simulink model "acf_detector_sl"  (R2018b)
settings: Solver=FixedStepDiscrete  StartTime=0.0  StopTime=inf  FixedStep=0.5  RelTol=1e-3
model workspace (MAT data in the model file):
  SL_ROS_VariableLengthArrays_MaxSizes.CommonInfo.ArrayTruncateAction = 'EmitWarning'
  SL_ROS_VariableLengthArrays_MaxSizes.MsgTypeMap = containers.Map
  SL_ROS_VariableLengthArrays_MaxSizes.MsgTypeMap.serialization.keys = {'autoware_msgs/image_obj', 'sensor_msgs/Image'}
  SL_ROS_VariableLengthArrays_MaxSizes.MsgTypeMap.serialization.values{1}(1).PropertyName = 'Obj'
  SL_ROS_VariableLengthArrays_MaxSizes.MsgTypeMap.serialization.values{1}(1).DataType = 'autoware_msgs/image_rect'
  SL_ROS_VariableLengthArrays_MaxSizes.MsgTypeMap.serialization.values{1}(1).MaxLength = 16
  SL_ROS_VariableLengthArrays_MaxSizes.MsgTypeMap.serialization.values{1}(2).PropertyName = 'Type'
  SL_ROS_VariableLengthArrays_MaxSizes.MsgTypeMap.serialization.values{1}(2).DataType = 'uint8'
  SL_ROS_VariableLengthArrays_MaxSizes.MsgTypeMap.serialization.values{1}(2).MaxLength = 128
  SL_ROS_VariableLengthArrays_MaxSizes.MsgTypeMap.serialization.values{2}(1).PropertyName = 'Data'
  SL_ROS_VariableLengthArrays_MaxSizes.MsgTypeMap.serialization.values{2}(1).DataType = 'uint8'
  SL_ROS_VariableLengthArrays_MaxSizes.MsgTypeMap.serialization.values{2}(1).MaxLength = 9560448
  SL_ROS_VariableLengthArrays_MaxSizes.MsgTypeMap.serialization.values{2}(2).PropertyName = 'Encoding'
  SL_ROS_VariableLengthArrays_MaxSizes.MsgTypeMap.serialization.values{2}(2).DataType = 'uint8'
  SL_ROS_VariableLengthArrays_MaxSizes.MsgTypeMap.serialization.values{2}(2).MaxLength = 128
  SL_ROS_VariableLengthArrays_MaxSizes.MsgTypeMap.serialization.uniformity = 0
  SL_ROS_VariableLengthArrays_MaxSizes.MsgTypeMap.serialization.keyType = 'char'
  SL_ROS_VariableLengthArrays_MaxSizes.MsgTypeMap.serialization.valueType = 'any'
undefined symbols (not defined in the file or in its folder): Header, Height, Label, Label_SL_Info, Objects, Objects_SL_Info, Score, Width, X, Y
libraries: robotlib x5
settings Model: Creator=handai  LastModifiedBy=sdd
settings DebuggingCC: LibraryContextMissingDiagnostic=none
settings SFSimCC: SimUseLocalCustomCode=off
settings RTWCC: RTWUseLocalCustomCode=off

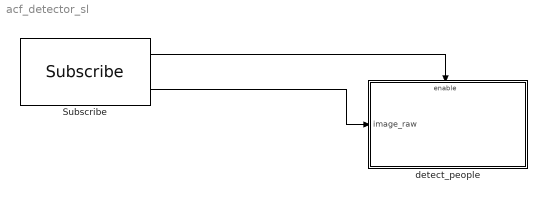
== system acf_detector_sl ==
  Subscribe : robotlib/Subscribe  topicSource=Specify your own  topic=/image_raw  messageType=sensor_msgs/Image  sampleTime=-1  messageQueueLength=1
      settings: SourceProductBaseCode=RO
  detect_people : Subsystem
  wires:
  Subscribe/1 -> detect_people/Enable
  Subscribe/2 -> detect_people/1(image_raw)

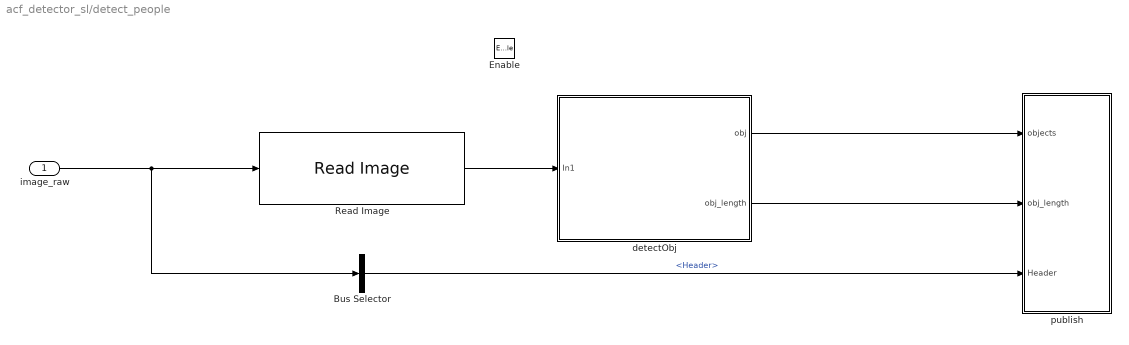
== system acf_detector_sl/detect_people ==
  image_raw : Inport
  Enable : EnablePort  PropagateVarSize=During execution
  Bus Selector : BusSelector  OutputSignals=Header
  Read Image : robotlib/Read Image  MaximumImageSize=[1544, 2064]  ImageEncoding=bgr8  ShowAlphaOutput=off  ShowErrorCodeOutput=off  VariableSizeOutputs=off
      settings: SourceProductName=Robotics System Toolbox  SourceProductBaseCode=RO
  detectObj : Subsystem
  publish : Subsystem
  wires:
  image_raw/1 -> Bus Selector/1, Read Image/1
  Read Image/1 -> detectObj/1(In1)
  detectObj/1(obj) -> publish/1(objects)
  detectObj/2(obj_length) -> publish/2(obj_length)
  Bus Selector/1 -> publish/3(Header)  "<Header>"

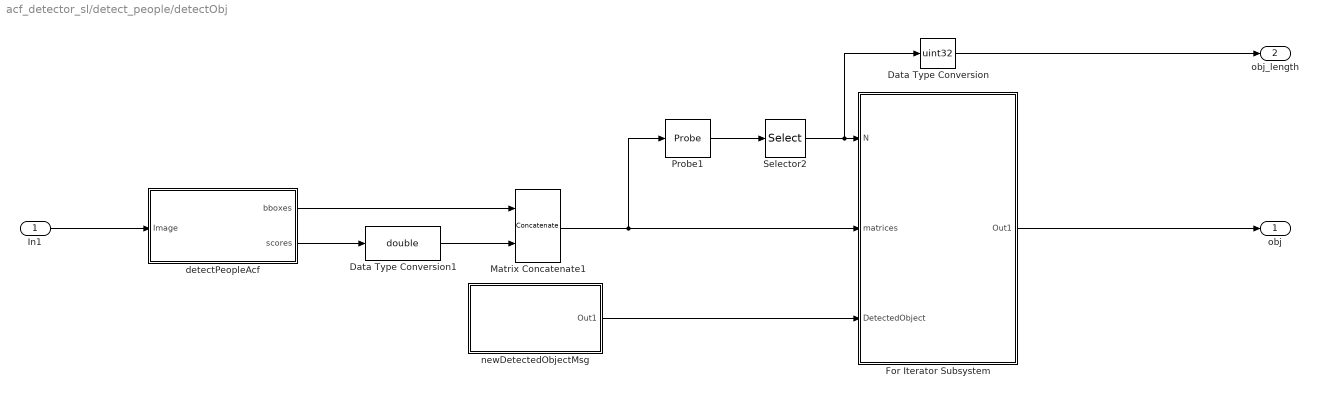
== system acf_detector_sl/detect_people/detectObj ==
  In1 : Inport
  Data Type Conversion : DataTypeConversion  OutDataTypeStr=uint32
  Data Type Conversion1 : DataTypeConversion  OutDataTypeStr=double
  For Iterator Subsystem : Subsystem  TreatAsAtomicUnit=on
  Matrix Concatenate1 : Concatenate  Mode=Multidimensional array  ConcatenateDimension=2
  Probe1 : Probe  ProbeWidth=off  ProbeSampleTime=off  ProbeComplexSignal=off  ProbeSignalDimensions=on
  Selector2 : Selector  InputPortWidth=2  IndexOptions=Index vector (dialog)  Indices=1  OutputSizes=1
  detectPeopleAcf : MATLAB Function  TreatAsAtomicUnit=on
  newDetectedObjectMsg : Subsystem
  obj : Outport
  obj_length : Outport  Port=2
  wires:
  detectPeopleAcf/1(bboxes) -> Matrix Concatenate1/1
  detectPeopleAcf/2(scores) -> Data Type Conversion1/1
  Selector2/1 -> Data Type Conversion/1, For Iterator Subsystem/1(N)
  In1/1 -> detectPeopleAcf/1(Image)
  newDetectedObjectMsg/1(Out1) -> For Iterator Subsystem/3(DetectedObject)
  For Iterator Subsystem/1(Out1) -> obj/1
  Probe1/1 -> Selector2/1
  Data Type Conversion1/1 -> Matrix Concatenate1/2
  Data Type Conversion/1 -> obj_length/1
  Matrix Concatenate1/1 -> For Iterator Subsystem/2(matrices), Probe1/1

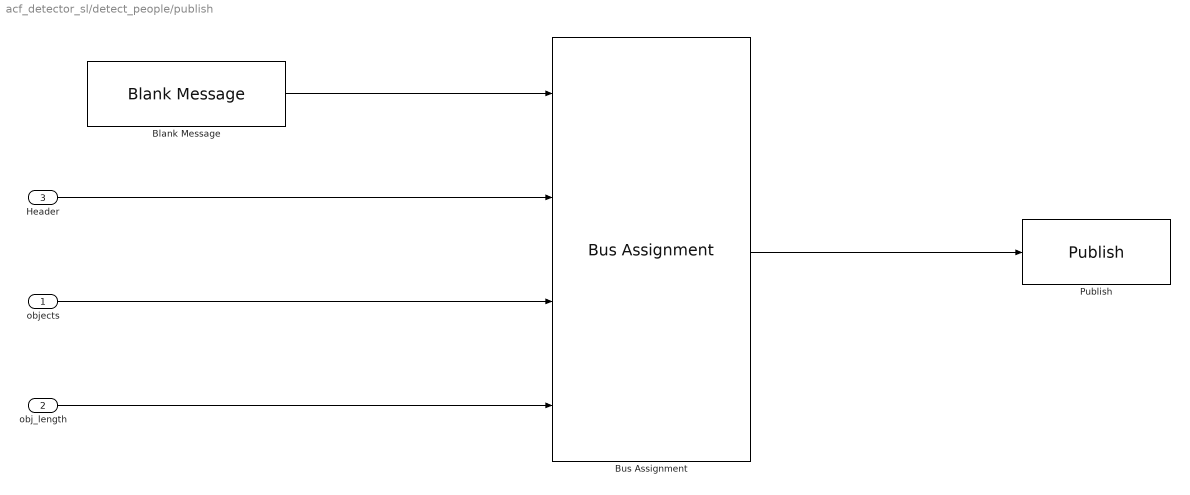
== system acf_detector_sl/detect_people/publish ==
  objects : Inport
  obj_length : Inport  Port=2
  Header : Inport  Port=3
  Blank Message : robotlib/Blank Message  messageClass=Message  entityType=autoware_msgs/DetectedObjectArray  messageType=autoware_msgs/DetectedObjectArray  SampleTime=inf
      settings: SourceProductBaseCode=RO
  Bus Assignment : BusAssignment  AssignedSignals=Header,Objects,Objects_SL_Info.CurrentLength
  Publish : robotlib/Publish  topicSource=Specify your own  topic=/detection/vision_objects  messageType=autoware_msgs/DetectedObjectArray  messageQueueLength=1
      settings: SourceProductBaseCode=RO
  wires:
  Bus Assignment/1 -> Publish/1
  Blank Message/1 -> Bus Assignment/1
  Header/1 -> Bus Assignment/2
  objects/1 -> Bus Assignment/3
  obj_length/1 -> Bus Assignment/4

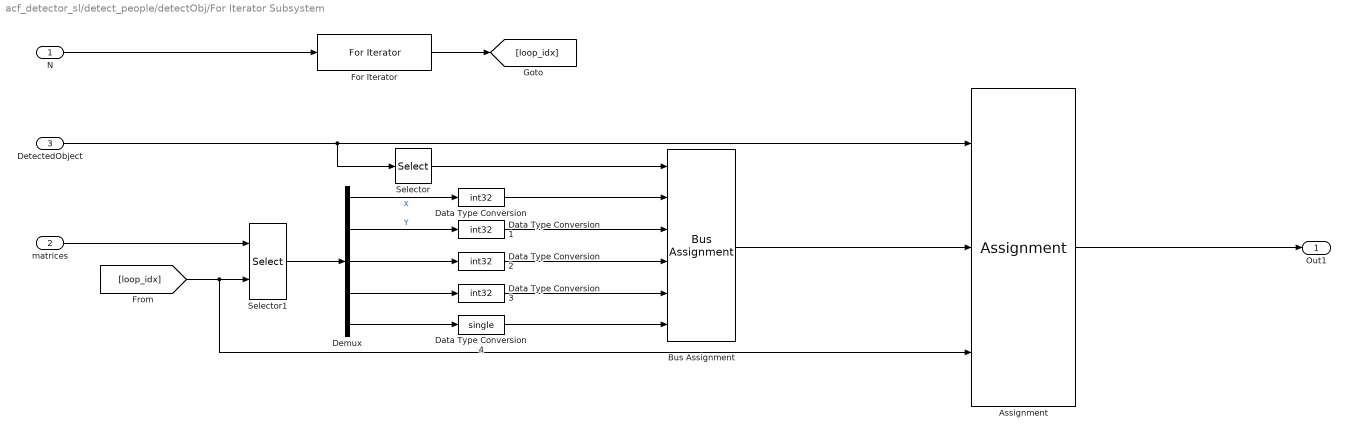
== system acf_detector_sl/detect_people/detectObj/For Iterator Subsystem ==
  N : Inport
  matrices : Inport  Port=2
  DetectedObject : Inport  Port=3
  Assignment : Assignment  DiagnosticForDimensions=Warning  IndexOptions=Index vector (port)  Indices=1  OutputSizes=1
  Bus Assignment : BusAssignment  AssignedSignals=X,Y,Width,Height,Score
  Data Type Conversion{,1..3} (4 alike) : DataTypeConversion  OutDataTypeStr=int32
  Data Type Conversion4 : DataTypeConversion  OutDataTypeStr=single
  Demux : Demux  Outputs=5
  For Iterator : ForIterator  ResetStates=reset  IterationSource=external
  Selector : Selector  InputPortWidth=16  IndexOptions=Index vector (dialog)  Indices=1  OutputSizes=1
  Selector1 : Selector  NumberOfDimensions=2  IndexOptions=Index vector (port),Index vector (dialog)  Indices=1,[1:5]  OutputSizes=1,1
  Out1 : Outport
  wires:
  Assignment/1 -> Out1/1
  DetectedObject/1 -> Selector/1, Assignment/1
  Selector1/1 -> Demux/1
  matrices/1 -> Selector1/1
  For Iterator/1 -> [loop_idx]
  [loop_idx] -> Assignment/3, Selector1/2
  N/1 -> For Iterator/1
  Selector/1 -> Bus Assignment/1
  Demux/3 -> Data Type Conversion2/1
  Demux/2 -> Data Type Conversion1/1  "Y"
  Demux/1 -> Data Type Conversion/1  "X"
  Demux/4 -> Data Type Conversion3/1
  Demux/5 -> Data Type Conversion4/1
  Data Type Conversion/1 -> Bus Assignment/2
  Data Type Conversion1/1 -> Bus Assignment/3
  Data Type Conversion2/1 -> Bus Assignment/4
  Data Type Conversion3/1 -> Bus Assignment/5
  Data Type Conversion4/1 -> Bus Assignment/6
  Bus Assignment/1 -> Assignment/2

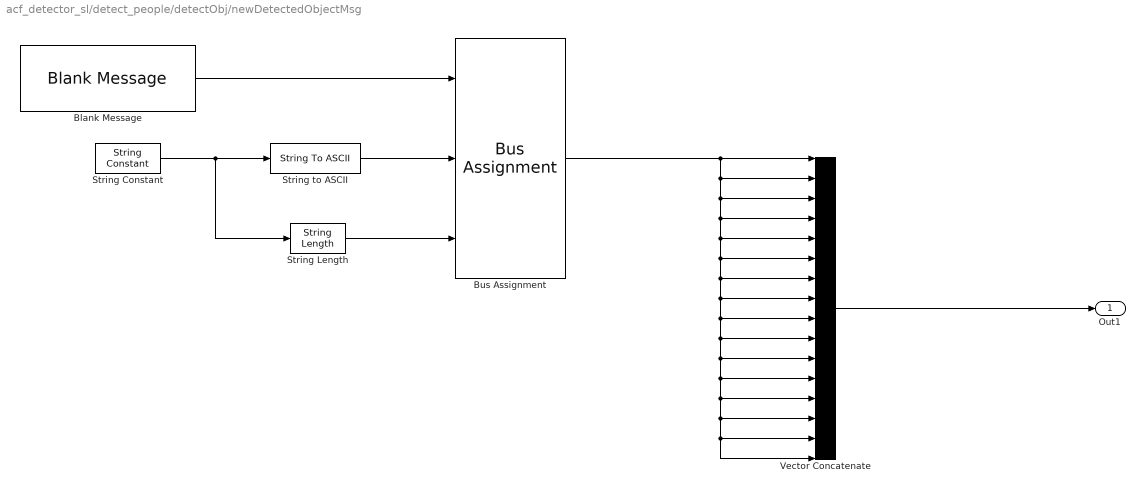
== system acf_detector_sl/detect_people/detectObj/newDetectedObjectMsg ==
  Blank Message : robotlib/Blank Message  messageClass=Message  entityType=autoware_msgs/DetectedObject  messageType=autoware_msgs/DetectedObject  SampleTime=inf
      settings: SourceProductBaseCode=RO
  Bus Assignment : BusAssignment  AssignedSignals=Label,Label_SL_Info.CurrentLength
  String Constant : StringConstant  String='Person'
  String Length : StringLength
  String to ASCII : StringToASCII  MaximumLength=128
  Vector Concatenate : Concatenate  NumInputs=16
  Out1 : Outport
  wires:
  Bus Assignment/1 -> Vector Concatenate/4, Vector Concatenate/6, Vector Concatenate/15, Vector Concatenate/16, Vector Concatenate/14, Vector Concatenate/13, Vector Concatenate/12, Vector Concatenate/11, Vector Concatenate/10, Vector Concatenate/9, Vector Concatenate/8, Vector Concatenate/7, Vector Concatenate/5, Vector Concatenate/3, Vector Concatenate/2, Vector Concatenate/1
  Vector Concatenate/1 -> Out1/1
  String Constant/1 -> String Length/1, String to ASCII/1
  Blank Message/1 -> Bus Assignment/1
  String to ASCII/1 -> Bus Assignment/2
  String Length/1 -> Bus Assignment/3

== matlab function acf_detector_sl/detect_people/detectObj/detectPeopleAcf ==
  settings: updateMethod=DISCRETE
  data: Image input; bboxes output size=[16 4]; scores output size=[16 1]
function [bboxes, scores] = detectPeopleAcf(Image)
coder.extrinsic('detectPeopleACF');
bboxes = zeros(16, 4);
scores = zeros(16, 1);
[bboxes, scores] = detectPeopleACF(Image);
